simulink model "ModelKinematicRobot"  (R2020b)
settings: Solver=FixedStepAuto  StartTime=0.0  StopTime=Inf  FixedStep=0.002  RelTol=1e-3
settings Model: Creator=kaebi  LastModifiedBy=kaebi
settings OptimizationCC: DefaultParameterBehavior=Inlined  LocalBlockOutputs=off
settings RTWCC: Description=TwinCAT GRT Target  SystemTargetFile=TwinCatGrt.tlc  GenCodeOnly=on  TemplateMakefile=tcgrt_msbuild.tmf  TargetLang=C++
settings STFCustomTargetCC: TargetLangStandard=C++03 (ISO)  ConcurrentExecutionCompliant=off  CombineOutputUpdateFcns=on  CodeInterfacePackaging=Reusable function  GRTInterface=off  GenerateAllocFcn=on  SystemTargetFile=TwinCatGrt.tlc
settings GRTTargetCC: TargetLangStandard=C++03 (ISO)  ParMdlRefBuildCompliant=off  CompOptLevelCompliant=off  ConcurrentExecutionCompliant=off  MatFileLogging=off  CodeInterfacePackaging=Reusable function  GenerateAllocFcn=on  UseToolchainInfoCompliant=off  ExtModeMexFile=TcExtModeClient

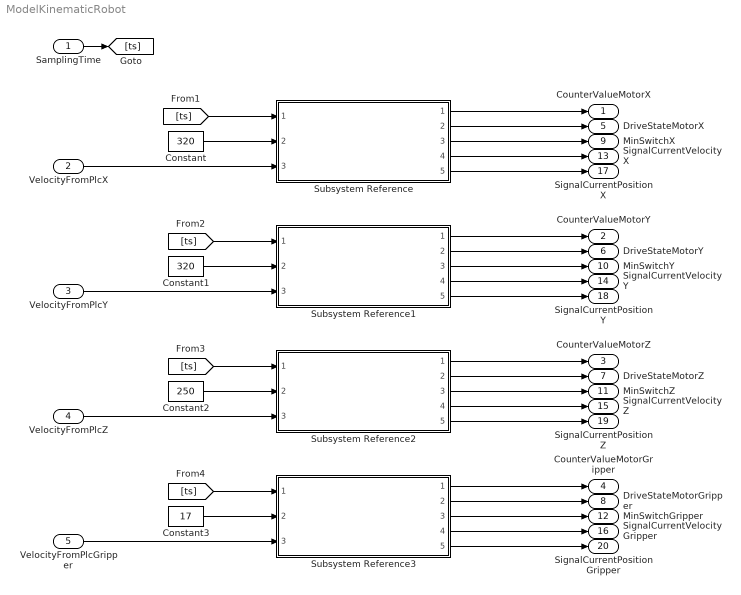
== system ModelKinematicRobot ==
  SamplingTime : Inport
  VelocityFromPlcX : Inport  Port=2  OutDataTypeStr=int16
  VelocityFromPlcY : Inport  Port=3  OutDataTypeStr=int16
  VelocityFromPlcZ : Inport  Port=4  OutDataTypeStr=int16
  VelocityFromPlcGripper : Inport  Port=5  OutDataTypeStr=int16
  Constant : Constant  Value=320
  Constant1 : Constant  Value=320
  Constant2 : Constant  Value=250
  Constant3 : Constant  Value=17
  Subsystem Reference{,1..3} (4 alike) : Subsystem  ReferencedSubsystem=SubSystemDrive
  CounterValueMotorX : Outport
  CounterValueMotorY : Outport  Port=2
  CounterValueMotorZ : Outport  Port=3
  CounterValueMotorGripper : Outport  Port=4
  DriveStateMotorX : Outport  Port=5
  DriveStateMotorY : Outport  Port=6
  DriveStateMotorZ : Outport  Port=7
  DriveStateMotorGripper : Outport  Port=8
  MinSwitchX : Outport  Port=9  OutDataTypeStr=boolean
  MinSwitchY : Outport  Port=10  OutDataTypeStr=boolean
  MinSwitchZ : Outport  Port=11  OutDataTypeStr=boolean
  MinSwitchGripper : Outport  Port=12  OutDataTypeStr=boolean
  SignalCurrentVelocityX : Outport  Port=13
  SignalCurrentVelocityY : Outport  Port=14
  SignalCurrentVelocityZ : Outport  Port=15
  SignalCurrentVelocityGripper : Outport  Port=16
  SignalCurrentPositionX : Outport  Port=17
  SignalCurrentPositionY : Outport  Port=18
  SignalCurrentPositionZ : Outport  Port=19
  SignalCurrentPositionGripper : Outport  Port=20
  wires:
  Subsystem Reference/4 -> SignalCurrentVelocityX/1
  Subsystem Reference/2 -> DriveStateMotorX/1
  Subsystem Reference/1 -> CounterValueMotorX/1
  SamplingTime/1 -> [ts]
  Constant/1 -> Subsystem Reference/2
  VelocityFromPlcZ/1 -> Subsystem Reference2/3
  VelocityFromPlcY/1 -> Subsystem Reference1/3
  VelocityFromPlcX/1 -> Subsystem Reference/3
  Constant1/1 -> Subsystem Reference1/2
  Constant2/1 -> Subsystem Reference2/2
  [ts] -> Subsystem Reference/1
  [ts] -> Subsystem Reference1/1
  [ts] -> Subsystem Reference2/1
  Subsystem Reference2/2 -> DriveStateMotorZ/1
  Subsystem Reference2/1 -> CounterValueMotorZ/1
  Subsystem Reference1/1 -> CounterValueMotorY/1
  Subsystem Reference1/2 -> DriveStateMotorY/1
  Subsystem Reference1/4 -> SignalCurrentVelocityY/1
  Subsystem Reference2/4 -> SignalCurrentVelocityZ/1
  Subsystem Reference2/5 -> SignalCurrentPositionZ/1
  Subsystem Reference1/5 -> SignalCurrentPositionY/1
  Subsystem Reference/5 -> SignalCurrentPositionX/1
  Subsystem Reference/3 -> MinSwitchX/1
  Subsystem Reference1/3 -> MinSwitchY/1
  Subsystem Reference2/3 -> MinSwitchZ/1
  Subsystem Reference3/3 -> MinSwitchGripper/1
  Subsystem Reference3/5 -> SignalCurrentPositionGripper/1
  Subsystem Reference3/4 -> SignalCurrentVelocityGripper/1
  Subsystem Reference3/1 -> CounterValueMotorGripper/1
  Subsystem Reference3/2 -> DriveStateMotorGripper/1
  [ts] -> Subsystem Reference3/1
  Constant3/1 -> Subsystem Reference3/2
  VelocityFromPlcGripper/1 -> Subsystem Reference3/3
